simulink model "RCAM_Model"  (R2022b)
settings: Solver=VariableStepAuto  StartTime=0.0  StopTime=TF  RelTol=1e-3
values from neighbouring files (symbols this model uses):
  U0 = [0 ... (first row only)    [RCAM_model_initialConditions.m]    (also in designPIL.m)
  X0 = [100 ... (first row only)    [RCAM_model_initialConditions.m]    (also in designPIL.m = [85)
libraries: sharedtransform x1
settings Model: Creator=bendr  LastModifiedBy=bendr

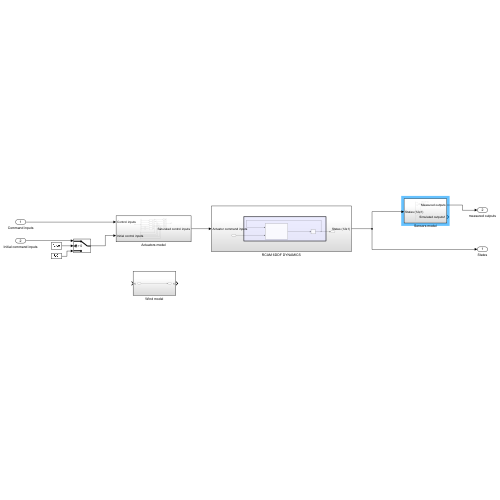
[thumbnail: Simulink's stored preview of the top-level diagram]
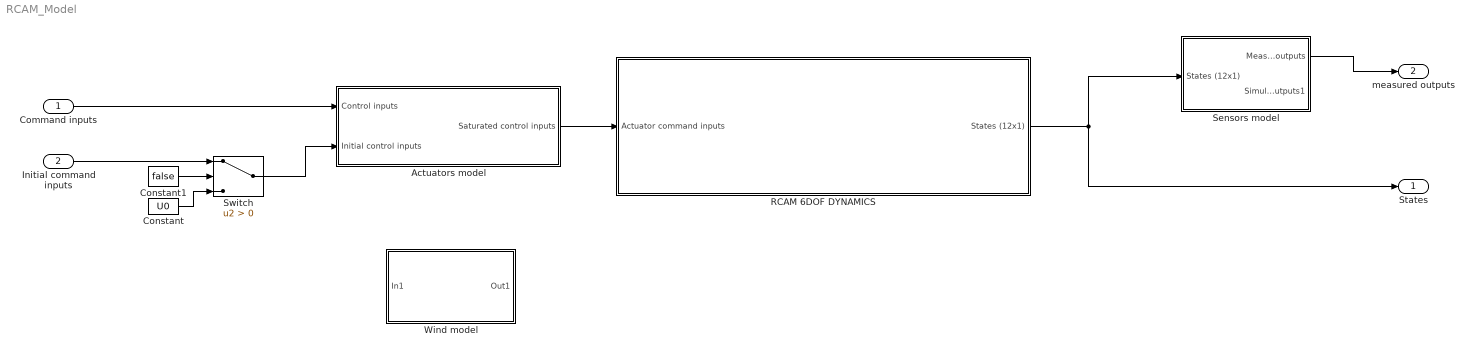
== system RCAM_Model ==
  Command inputs : Inport
  Initial command inputs : Inport  Port=2
  Actuators model : Subsystem
  Constant : Constant  Value=U0
  Constant1 : Constant  Value=false
  RCAM 6DOF DYNAMICS : Subsystem
  Sensors model : Subsystem
  Switch : Switch  Criteria=u2 > Threshold  SaturateOnIntegerOverflow=off  InputSameDT=off
  Wind model : Subsystem
  States : Outport
  measured outputs : Outport  Port=2
  wires:
  RCAM 6DOF DYNAMICS/1(States (12x1)) -> Sensors model/1(States (12x1)), States/1
  Constant1/1 -> Switch/2
  Initial command inputs/1 -> Switch/1
  Constant/1 -> Switch/3
  Command inputs/1 -> Actuators model/1(Control inputs)
  Actuators model/1(Saturated control inputs) -> RCAM 6DOF DYNAMICS/1(Actuator command inputs)
  Sensors model/1(Measured outputs) -> measured outputs/1
  Switch/1 -> Actuators model/2(Initial control inputs)

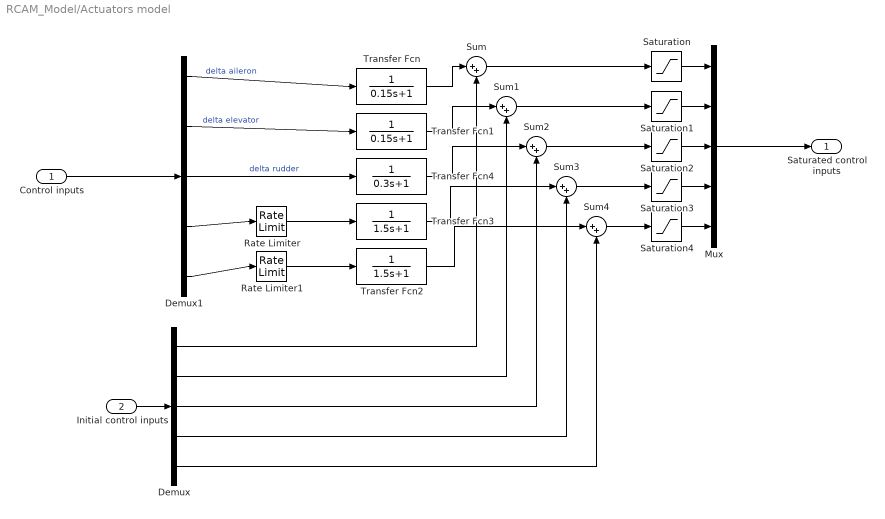
== system RCAM_Model/Actuators model ==
  Control inputs : Inport
  Initial control inputs : Inport  Port=2
  Demux : Demux  Outputs=5
  Demux1 : Demux  Outputs=5
  Mux : Mux  Inputs=5
  Rate Limiter : RateLimiter  RisingSlewLimit=1.6  FallingSlewLimit=-1.6  SampleTimeMode=inherited
  Rate Limiter1 : RateLimiter  RisingSlewLimit=1.6  FallingSlewLimit=-1.6  SampleTimeMode=inherited
  Saturation : Saturate  UpperLimit=25  LowerLimit=-25
  Saturation1 : Saturate  UpperLimit=10  LowerLimit=-25
  Saturation2 : Saturate  UpperLimit=30  LowerLimit=-30
  Saturation3 : Saturate  UpperLimit=1  LowerLimit=0.5
  Saturation4 : Saturate  UpperLimit=1  LowerLimit=0.5
  Sum{,1..4} (5 alike) : Sum  Inputs=|++
  Transfer Fcn : TransferFcn  Denominator=[0.15 1]
  Transfer Fcn1 : TransferFcn  Denominator=[0.15 1]
  Transfer Fcn2 : TransferFcn  Denominator=[1.5 1]
  Transfer Fcn3 : TransferFcn  Denominator=[1.5 1]
  Transfer Fcn4 : TransferFcn  Denominator=[0.3 1]
  Saturated control inputs : Outport
  wires:
  Initial control inputs/1 -> Demux/1
  Control inputs/1 -> Demux1/1
  Demux1/4 -> Rate Limiter/1
  Demux1/5 -> Rate Limiter1/1
  Mux/1 -> Saturated control inputs/1
  Demux/1 -> Sum/2
  Demux/2 -> Sum1/2
  Demux/3 -> Sum2/2
  Demux/4 -> Sum3/2
  Demux/5 -> Sum4/2
  Transfer Fcn/1 -> Sum/1
  Demux1/1 -> Transfer Fcn/1  "delta aileron"
  Demux1/2 -> Transfer Fcn1/1  "delta elevator"
  Demux1/3 -> Transfer Fcn4/1  "delta rudder"
  Rate Limiter/1 -> Transfer Fcn3/1
  Rate Limiter1/1 -> Transfer Fcn2/1
  Transfer Fcn1/1 -> Sum1/1
  Transfer Fcn4/1 -> Sum2/1
  Transfer Fcn3/1 -> Sum3/1
  Transfer Fcn2/1 -> Sum4/1
  Saturation/1 -> Mux/1
  Saturation1/1 -> Mux/2
  Saturation2/1 -> Mux/3
  Saturation3/1 -> Mux/4
  Saturation4/1 -> Mux/5
  Sum/1 -> Saturation/1
  Sum1/1 -> Saturation1/1
  Sum2/1 -> Saturation2/1
  Sum3/1 -> Saturation3/1
  Sum4/1 -> Saturation4/1

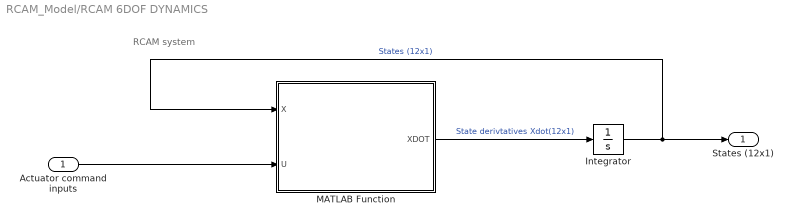
== system RCAM_Model/RCAM 6DOF DYNAMICS ==
  note: RCAM system
  Actuator command inputs : Inport
  Integrator : Integrator  InitialCondition=X0  ContinuousStateAttributes={'u','v','w','p','q','r','phi','theta','psi','XNED','YNED','ZNED'}
  MATLAB Function : MATLAB Function  TreatAsAtomicUnit=on
  States (12x1) : Outport
  wires:
  Integrator/1 -> States (12x1)/1, MATLAB Function/1(X)  "States (12x1)"
  Actuator command inputs/1 -> MATLAB Function/2(U)
  MATLAB Function/1(XDOT) -> Integrator/1  "State derivtatives Xdot(12x1)"

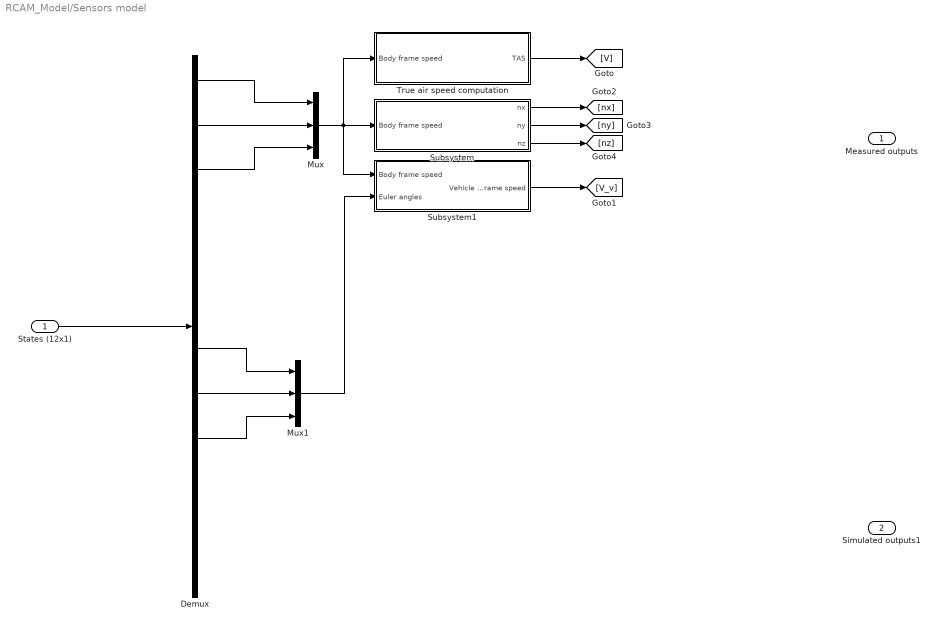
== system RCAM_Model/Sensors model ==
  States (12x1) : Inport
  Demux : Demux  Outputs=12
  Mux : Mux  Inputs=3
  Mux1 : Mux  Inputs=3
  Subsystem : Subsystem
  Subsystem1 : Subsystem
  True air speed computation : Subsystem
  Measured outputs : Outport
  Simulated outputs1 : Outport  Port=2
  wires:
  States (12x1)/1 -> Demux/1
  Mux/1 -> True air speed computation/1(Body frame speed), Subsystem1/1(Body frame speed), Subsystem/1(Body frame speed)
  Demux/1 -> Mux/1
  Demux/2 -> Mux/2
  Demux/3 -> Mux/3
  True air speed computation/1(TAS) -> [V]
  Demux/8 -> Mux1/2
  Demux/7 -> Mux1/1
  Demux/9 -> Mux1/3
  Mux1/1 -> Subsystem1/2(Euler angles)
  Subsystem1/1(Vehicle frame speed) -> [V_v]
  Subsystem/1(nx) -> [nx]
  Subsystem/2(ny) -> [ny]
  Subsystem/3(nz) -> [nz]

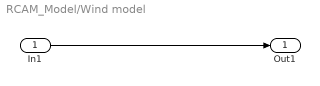
== system RCAM_Model/Wind model ==
  In1 : Inport
  Out1 : Outport
  wires:
  In1/1 -> Out1/1

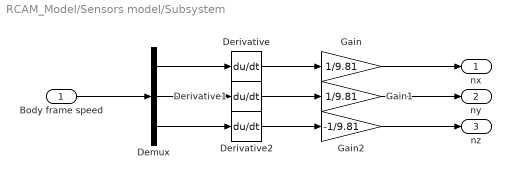
== system RCAM_Model/Sensors model/Subsystem ==
  Body frame speed : Inport
  Demux : Demux  Outputs=3
  Derivative : Derivative
  Derivative1 : Derivative
  Derivative2 : Derivative
  Gain : Gain  Gain=1/9.81
  Gain1 : Gain  Gain=1/9.81
  Gain2 : Gain  Gain=-1/9.81
  nx : Outport
  ny : Outport  Port=2
  nz : Outport  Port=3
  wires:
  Body frame speed/1 -> Demux/1
  Demux/1 -> Derivative/1
  Demux/2 -> Derivative1/1
  Demux/3 -> Derivative2/1
  Derivative/1 -> Gain/1
  Derivative1/1 -> Gain1/1
  Derivative2/1 -> Gain2/1
  Gain/1 -> nx/1
  Gain1/1 -> ny/1
  Gain2/1 -> nz/1

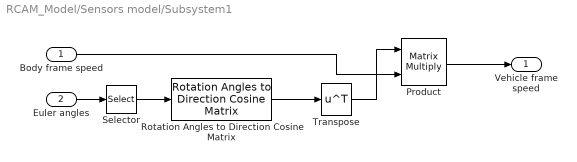
== system RCAM_Model/Sensors model/Subsystem1 ==
  Body frame speed : Inport
  Euler angles : Inport  Port=2
  Product : Product  Multiplication=Matrix(*)
  Rotation Angles to Direction Cosine Matrix : sharedtransform/Rotation Angles to Direction Cosine Matrix  rotationOrder=ZYX  aMode=aMode
  Selector : Selector  InputPortWidth=3  IndexOptions=Index vector (dialog)  Indices=[3 2 1]  OutputSizes=1
  Transpose : Math  Operator=transpose
  Vehicle frame speed : Outport
  wires:
  Selector/1 -> Rotation Angles to Direction Cosine Matrix/1
  Euler angles/1 -> Selector/1
  Rotation Angles to Direction Cosine Matrix/1 -> Transpose/1
  Product/1 -> Vehicle frame speed/1
  Body frame speed/1 -> Product/2
  Transpose/1 -> Product/1

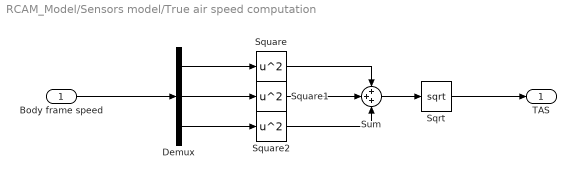
== system RCAM_Model/Sensors model/True air speed computation ==
  Body frame speed : Inport
  Demux : Demux  Outputs=3
  Sqrt : Sqrt
  Square : Math  Operator=square
  Square1 : Math  Operator=square
  Square2 : Math  Operator=square
  Sum : Sum  Inputs=+++
  TAS : Outport
  wires:
  Body frame speed/1 -> Demux/1
  Demux/1 -> Square/1
  Demux/2 -> Square1/1
  Demux/3 -> Square2/1
  Square1/1 -> Sum/2
  Square/1 -> Sum/1
  Square2/1 -> Sum/3
  Sum/1 -> Sqrt/1
  Sqrt/1 -> TAS/1

== matlab function RCAM_Model/RCAM 6DOF DYNAMICS/MATLAB Function ==
  data: X input; XDOT output; U input
function XDOT  = RCAM_model(X,U)

%-----------STATE AND CONTROL VECTORS-------------

x1 = X(1); %u
x2 = X(2); %v
x3 = X(3); %w
x4 = X(4); %p
x5 = X(5); %q
x6 = X(6); %r
x7 = X(7); %phi
x8 = X(8); %theta
x9 = X(9); %psi
x10 = X(10); % X position in Earth frame of reference.
x11 = X(11); % Y position in Earth frame of reference.
x12 = X(12); % Z position in Earth frame of reference.

u1 = U(1); %d_A (Aileron)
u2 = U(2); %d_T (Stabilizer)
u3 = U(3); %d_R (Rudder)
u4 = U(4); %d_th1 (throttle 1)
u5 = U(5); %d_th2 (throttle 2)

%-----------CONSTANTS------------------------------

m = 120000; % Aircraft mass (Kg)

cbar = 6.6; % Mean Aerodynamic Chord (m)
lt = 24.8;  % Distance of AC of tail and body (m)
S = 260;    % Wing planform area (m^2)
St = 64;    % Tail planform area (m^2)

Xcg = 0.23*cbar;  % x position of CG in Fm (m)
Ycg = 0;          % y position of CG in Fm (m)
Zcg = 0.1*cbar;   % z position of CG in Fm (m)

Xac = 0.12*cbar;  % x position of Aerodynamic Center in Fm (m)
Yac = 0;          % y position of Aerodynamic Center in Fm (m)
Zac = 0;          % z position of Aerodynamic Center in Fm (m)

%Engine constants

Xapt1 = 0;        % x position of engine 1 force in Fm (m)
Yapt1 = -7.94;    % y position of engine 1 force in Fm (m)
Zapt1 = -1.9;     % z position of engine 1 force in Fm (m)

Xapt2 = 0;        % x position of engine 2 force in Fm (m)
Yapt2 = 7.94;     % y position of engine 2 force in Fm (m)
Zapt2 = -1.9;     % z position of engine 2 force in Fm (m)

%Other constants
rho = 1.225;
g = 9.81;
depsda = 0.25;           % Change in downwash w.r.t. alpha (rad/rad)
alpha_L0 = -11.5*pi/180; % Zero lift AOA (rad)
n= 5.5;                  % Slope of linear region of lift slope
a3 = -768.5;             % Coefficient of alpha^3
a2 = 609.2;              % Coefficient of alpha^2
a1 = -155.2;             % Coefficient of alpha^1
a0 = 15.212;             % Coefficient of alpha^0
alpha_switch = 14.5*(pi/180); % alpha where lift slope goes from linear to non-linear

%-----------CONTROL LIMITS SATURATION------------------------------

u1min = -25*pi/180;
u1max =  25*pi/180;

u2min = -25*pi/180;
u2max =  10*pi/180;

u3min = -30*pi/180;
u3max =  30*pi/180;

u4min =  0.5*pi/180;
u4max =  10*pi/180;

u5min =  0.5*pi/180;
u5max =  10*pi/180;

if(u1>u1max)
    u1=u1max;
elseif(u1<u1min)
    u1=u1min;
end

if(u2>u2max)
    u2=u2max;
elseif(u2<u2min)
    u2=u2min;
end

if(u3>u3max)
    u3=u3max;
elseif(u3<u3min)
    u3=u3min;
end

if(u4>u4max)
    u4=u4max;
elseif(u4<u4min)
    u4=u4min;
end

if(u5>u5max)
    u5=u5max;
elseif(u5<u5min)
    u5=u5min;
end

%-------------INTERMEDIATE VARIABLES-----------------------------

Va = sqrt(x1^2+ x2^2 +x3^2);   %airspeed

alpha = atan2(x3,x1); % alpha
beta = asin(x2/Va);   %beta

Q = 0.5*rho*Va^2;     %dynamic pressure

wbe_b = [x4;x5;x6];
V_b = [x1;x2;x3];

%--------------Aerodynamic Force Coefficients---------------------

%CL_wingbody
if alpha<=alpha_switch
    CL_wb = n*(alpha -alpha_L0);
else
    CL_wb = a3*alpha^3 + a2*alpha^2 + a1*alpha + a0;
end

%CL_tail
epsilon = depsda*(alpha - alpha_L0);
alpha_t = alpha - epsilon + u2 + 1.3*x5*lt/Va;
CL_t = 3.1*(St/S)*alpha_t;

%Total Lift coefficient
CL = CL_wb + CL_t;

%Total Drag force
CD = 0.13 + 0.07*(5.5*alpha + 0.654)^2;

%Side forces
CY = -1.6*beta + 0.24*u3;

%------------------------4. Dimensional Aero Forces--------------------

% Actual dimensional forces in F_s (Stability axis)

FA_s = [-CD*Q*S;
         CY*Q*S;
        -CL*Q*S];

% Rotate forces to F_b (body axis)

C_bs = [cos(alpha) 0 -sin(alpha);0 1 0;sin(alpha) 0 cos(alpha)];   % rotation matrix

FA_b = C_bs*FA_s;

%------------------------5. Aero Moment Coefficient about AC--------------
%calculate moments in F_b

eta11 = -1.4*beta;
eta21 = -0.59 - (3.1*(St*lt)/(S*cbar))*(alpha - epsilon);
eta31 = (1-alpha*(180/(15*pi)))*beta;

eta = [eta11;eta21;eta31];

dCMdx = (cbar/Va)*[-11 0 5;0 (-4.03*(St*lt^2)/(S*cbar^2)) 0;1.7 0 -11.5];

dCMdu = [-0.6 0 0.22;0 (-3.1*(St*lt)/(S*cbar)) 0;0 0 -0.63];

% CM = [Cl;Cm;Cn] about Aero center in F_b
CMac_b = eta + dCMdx*wbe_b + dCMdu*[u1;u2;u3];

%-------------------------6. Aero moment about AC--------------------------
% Normalize to an aero moment
MAac_b = CMac_b*Q*S*cbar;

%-------------------------7. Aero moment about CG--------------------------
%transfer monet to CG
rcg_b = [Xcg;Ycg;Zcg];
rac_b = [Xac;Yac;Zac];
MAcg_b = MAac_b + cross(FA_b,rcg_b - rac_b);

%-------------------------8. Engine Force & Moment-------------------------
T2W = 0.35; % Thrust to weight ratio
F1=u4*T2W*m*g;
F2=u5*T2W*m*g;

%Assuming engine thrust is aligned with body frame

FE1_b = [F1;
        0;
        0];
FE2_b = [F2;
        0;
        0];

FE_b = FE1_b + FE2_b;

%Now engine moment due to offset of thrust from CG

mew1 = [Xcg-Xapt1;
        Yapt1-Ycg;
        Zcg-Zapt1];
    
mew2 = [Xcg-Xapt2;
        Yapt2-Ycg;
        Zcg-Zapt2];
    
MEcg1_b = cross(mew1,FE1_b);
MEcg2_b = cross(mew2,FE2_b);

MEcg_b = MEcg1_b + MEcg2_b;

%----------------------------9. Gravity Effect-----------------------------
%Calculate gravitational forces in body frame. This causes no moment
%about--cg

g_b = [-g*sin(x8);g*cos(x8)*sin(x7);g*cos(x8)*cos(x7)];

Fg_b = m*g_b;

%----------------------------10. State Derivatives------------------------

%Inertia Matrix

Ib = m*[40.07 0 -2.0923;
        0 64 0;
        -2.0923 0 99.92];

invIb = (1/m)*[0.0249836 0 0.000523151;
               0 0.015625 0;
               0.000523151 0 0.010019];
           
F_b = Fg_b + FE_b + FA_b;
x1to3dot = (1/m)*F_b - cross(wbe_b,V_b);

Mcg_b = MAcg_b + MEcg_b;
x4to6dot = invIb*(Mcg_b - cross(wbe_b,Ib*wbe_b));

H_phi = [1 sin(x7)*tan(x8) cos(x7)*tan(x8);
         0 cos(x7) -sin(x7);
         0 sin(x7)/cos(x8) cos(x7)/cos(x8)];
     
x7to9dot = H_phi*wbe_b;

% Rotation matrices:

R_theta = [cos(x8) 0 -sin(x8); 0 1 0; sin(x8) 0 cos(x8)];
R_phi = [1 0 0; 0 cos(x7) -sin(x7); 0 sin(x7) cos(x7)];
R_psi = [cos(x9) -sin(x9) 0; sin(x9) cos(x9) 0; 0 0 1];

R_B2V = R_phi*R_theta*R_psi;
R_V2B = R_B2V';

% XYZ derivatives in Earth reference frame:

x10to12dot = R_V2B*[x1;x2;x3];

%Place in first order form


XDOT = [x1to3dot;
        x4to6dot;
        x7to9dot;
        x10to12dot];
end
